simulink model "BatchEventsFor3StateMachines"  (R2021b)
settings: Solver=VariableStepAuto  StartTime=0.0  StopTime=10.0  RelTol=1e-3
model workspace (MATLAB code in the model file):
  | % Add the class folders into the path.
  | addpath model
  | addpath utils
  | 
  | %% Loading data from files.
  | % Data for supervisor 1.
  | utils1 = StateMachineUtils;
  | 
  | % From TCT: Load all events' number.
  | utils1 = utils1.loadEventsInAds('resources/tct/ALLEVENT.ADS');
  | 
  | % From TCT: Disabled events in each state.
  | utils1 = utils1.loadDisabledEventsInPdt('resources/tct/supervisor1/DATA_SIMSUP1_MG1.PDT');
  | 
  | % From TCT: Transition matrix.
  | utils1 = utils1.loadTransitionsInAds('resources/tct/supervisor1/SIMSUP1_MG1.ADS');
  | 
  | % Parameters for the block.
  | encodedStates1 = StateEncoder.encode(utils1.statesArray);
  | 
  | transitions1 = utils1.transitions;
  | 
  | allEvents1 = utils1.eventsArray;
  | 
  | % Data for supervisor 2.
  | utils2 = StateMachineUtils;
  | 
  | % From TCT: Load all events' number.
  | utils2 = utils2.loadEventsInAds('resources/tct/ALLEVENT.ADS');
  | 
  | % From TCT: Disabled events in each state.
  | utils2 = utils2.loadDisabledEventsInPdt('resources/tct/supervisor2/DATA_SIMSUP2_MG1.PDT');
  | 
  | % From TCT: Transition matrix.
  | utils2 = utils2.loadTransitionsInAds('resources/tct/supervisor2/SIMSUP2_MG1.ADS');
  | 
  | % Parameters for the block.
  | encodedStates2 = StateEncoder.encode(utils2.statesArray);
  | 
  | transitions2 = utils2.transitions;
  | 
  | allEvents2 = utils2.eventsArray;
  | 
  | % Data for supervisor 3.
  | utils3 = StateMachineUtils;
  | 
  | % From TCT: Load all events' number.
  | utils3 = utils3.loadEventsInAds('resources/tct/ALLEVENT.ADS');
  | 
  | % From TCT: Disabled events in each state.
  | utils3 = utils3.loadDisabledEventsInPdt('resources/tct/supervisor3/DATA_SIMSUP3_MG1.PDT');
  | 
  | % From TCT: Transition matrix.
  | utils3 = utils3.loadTransitionsInAds('resources/tct/supervisor3/SIMSUP3_MG1.ADS');
  | 
  | % Parameters for the block.
  | encodedStates3 = StateEncoder.encode(utils3.statesArray);
  | 
  | transitions3 = utils3.transitions;
  | 
  | allEvents3 = utils3.eventsArray;
settings Model: Creator=andrerangel  LastModifiedBy=andrerangel

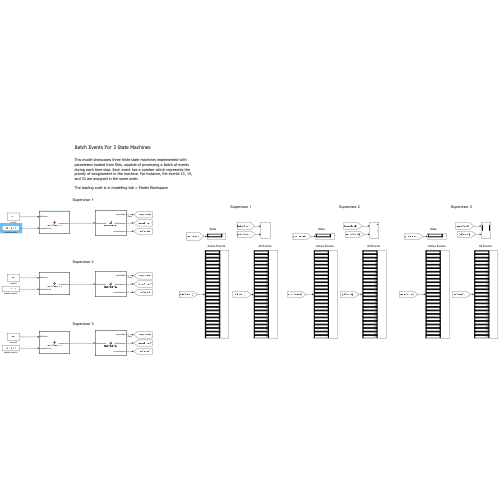
[thumbnail: Simulink's stored preview of the top-level diagram]
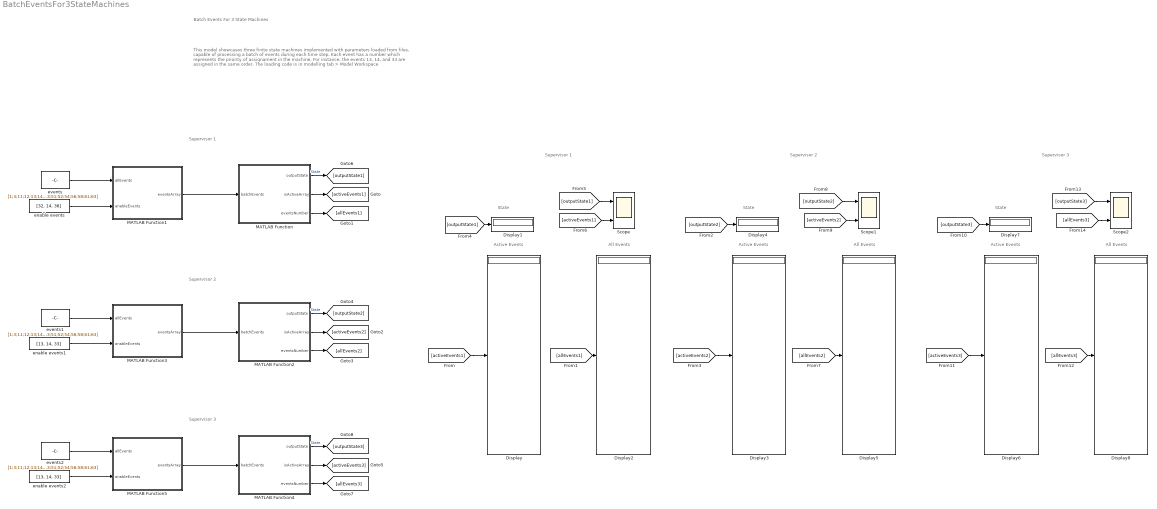
== system BatchEventsFor3StateMachines ==
  note: Active Events
  note: State
  note: This model showcases three finite state machines implemented with parameters loaded from files, capable of processing a batch of events during each time step. Each event has a number which represents the priority of assignament in the machine. For instance, the events 13, 14, and 33 are assigned in the same order.
      |
      | The loading code is in modelling tab > Model Workspace
  note: Supervisor 1
  note: All Events
  note: Batch Events For 3 State Machines
  note: All Events
  note: Supervisor 2
  note: Active Events
  note: State
  note: Supervisor 1
  note: All Events
  note: Supervisor 3
  note: Active Events
  note: State
  note: Supervisor 2
  note: Supervisor 3
  Display{,1..8} (9 alike) : Display
  MATLAB Function : MATLAB Function  TreatAsAtomicUnit=on
  MATLAB Function1 : MATLAB Function  TreatAsAtomicUnit=on
  MATLAB Function2 : MATLAB Function  TreatAsAtomicUnit=on
  MATLAB Function3 : MATLAB Function  TreatAsAtomicUnit=on
  MATLAB Function4 : MATLAB Function  TreatAsAtomicUnit=on
  MATLAB Function5 : MATLAB Function  TreatAsAtomicUnit=on
  Scope : Scope  NumInputPorts=2
  Scope1 : Scope  NumInputPorts=2
  Scope2 : Scope  NumInputPorts=2
  enable events : Constant  Value=[32, 14, 36]
  enable events1 : Constant  Value=[13, 14, 33]
  enable events2 : Constant  Value=[13, 14, 33]
  events : Constant  Value=[1;3;11;12;13;14;16;21;23;25;27;31;32;33;34;36;41;43;51;52;54;56;58;61;63]
  events1 : Constant  Value=[1;3;11;12;13;14;16;21;23;25;27;31;32;33;34;36;41;43;51;52;54;56;58;61;63]
  events2 : Constant  Value=[1;3;11;12;13;14;16;21;23;25;27;31;32;33;34;36;41;43;51;52;54;56;58;61;63]
  wires:
  MATLAB Function1/1(eventsArray) -> MATLAB Function/1(batchEvents)
  [allEvents1] -> Display2/1
  [outputState2] -> Scope1/1
  [allEvents2] -> Display5/1
  [activeEvents2] -> Scope1/2
  [activeEvents2] -> Display3/1
  MATLAB Function/1(outputState) -> [outputState1]  "State"
  enable events/1 -> MATLAB Function1/2(anableEvents)
  [outputState1] -> Display1/1
  events/1 -> MATLAB Function1/1(allEvents)
  [activeEvents1] -> Scope/2
  [outputState1] -> Scope/1
  [outputState2] -> Display4/1
  MATLAB Function/2(isActiveArray) -> [activeEvents1]
  [activeEvents1] -> Display/1
  MATLAB Function/3(eventsNumber) -> [allEvents1]
  MATLAB Function2/3(eventsNumber) -> [allEvents2]
  MATLAB Function2/2(isActiveArray) -> [activeEvents2]
  events1/1 -> MATLAB Function3/1(allEvents)
  enable events1/1 -> MATLAB Function3/2(anableEvents)
  MATLAB Function2/1(outputState) -> [outputState2]  "State"
  MATLAB Function3/1(eventsArray) -> MATLAB Function2/1(batchEvents)
  MATLAB Function5/1(eventsArray) -> MATLAB Function4/1(batchEvents)
  MATLAB Function4/1(outputState) -> [outputState3]  "State"
  enable events2/1 -> MATLAB Function5/2(anableEvents)
  events2/1 -> MATLAB Function5/1(allEvents)
  MATLAB Function4/2(isActiveArray) -> [activeEvents3]
  MATLAB Function4/3(eventsNumber) -> [allEvents3]
  [outputState3] -> Display7/1
  [activeEvents3] -> Display6/1
  [allEvents3] -> Scope2/2
  [allEvents3] -> Display8/1
  [outputState3] -> Scope2/1

== matlab function BatchEventsFor3StateMachines/MATLAB Function1 ==
  data: allEvents input; anableEvents input; eventsArray output
function eventsArray = eventsGenerator(allEvents, anableEvents)

[~, indexes] = ismember(anableEvents, allEvents);

eventsArray = zeros(length(allEvents), 1);

eventsArray(indexes) = 1;

== matlab function BatchEventsFor3StateMachines/MATLAB Function ==
  data: batchEvents input; outputState output size=[1 1]; isActiveArray output; eventsNumber output; allEvents1 parameter; transitions1 parameter; encodedStates1 parameter
function [outputState, isActiveArray, eventsNumber] = stateMachine1( ...
    batchEvents, ...
    allEvents1, ...
    transitions1, ...
    encodedStates1)
% State Machine with parameters from files.
% Receives a batch of events and process one event at time, starting with
% the event of index 1.
% batchEvents: array with 0s and 1s where 1 is the enabled event while 0,
% is disabled event;
% allEvents: numbers of the events;
% transitions: matrix of transitions;
% encodedStates: Encoded states array to be decoded before the pass it to
% StateMachines as an argument.

% Initialize a persistent object. Its value will not be erased as this
% block finishes.
persistent stateMachine

% Assign the persistent object to the StateMachine class with data passed
% as parameters.
if (isempty(stateMachine))
    statesArray = StateEncoder.decode(encodedStates1);                        
    stateMachine = StateMachine(statesArray, transitions1, allEvents1);
end

anabledEvents = allEvents1(logical(batchEvents));

% loop through an array of events:
for i=1:length(anabledEvents)
    stateMachine.inputEvent = anabledEvents(i);
end
outputState = stateMachine.currentState.number;
isActiveArray = stateMachine.currentState.activeEvents;
eventsNumber = stateMachine.eventsArray;

== matlab function BatchEventsFor3StateMachines/MATLAB Function2 ==
  data: batchEvents input; outputState output size=[1 1]; isActiveArray output; eventsNumber output; allEvents2 parameter; transitions2 parameter; encodedStates2 parameter
function [outputState, isActiveArray, eventsNumber] = stateMachine2( ...
    batchEvents, ...
    allEvents2, ...
    transitions2, ...
    encodedStates2)
% State Machine with parameters from files.
% Receives a batch of events and process one event at time, starting with
% the event of index 1.
% batchEvents: array with 0s and 1s where 1 is the enabled event while 0,
% is disabled event;
% allEvents: numbers of the events;
% transitions: matrix of transitions;
% encodedStates: Encoded states array to be decoded before the pass it to
% StateMachines as an argument.

% Initialize a persistent object. Its value will not be erased as this
% block finishes.
persistent stateMachine

% Assign the persistent object to the StateMachine class with data passed
% as parameters.
if (isempty(stateMachine))
    statesArray = StateEncoder.decode(encodedStates2);                        
    stateMachine = StateMachine(statesArray, transitions2, allEvents2);
end

anabledEvents = allEvents2(logical(batchEvents));

% loop through an array of events:
for i=1:length(anabledEvents)
    stateMachine.inputEvent = anabledEvents(i);
end
outputState = stateMachine.currentState.number;
isActiveArray = stateMachine.currentState.activeEvents;
eventsNumber = stateMachine.eventsArray;

== matlab function BatchEventsFor3StateMachines/MATLAB Function3 ==
  data: allEvents input; anableEvents input; eventsArray output
function eventsArray = eventsGenerator(allEvents, anableEvents)

[~, indexes] = ismember(anableEvents, allEvents);

eventsArray = zeros(length(allEvents), 1);

eventsArray(indexes) = 1;

== matlab function BatchEventsFor3StateMachines/MATLAB Function4 ==
  data: batchEvents input; outputState output size=[1 1]; isActiveArray output; eventsNumber output; allEvents3 parameter; transitions3 parameter; encodedStates3 parameter
function [outputState, isActiveArray, eventsNumber] = stateMachine3( ...
    batchEvents, ...
    allEvents3, ...
    transitions3, ...
    encodedStates3)
% State Machine with parameters from files.
% Receives a batch of events and process one event at time, starting with
% the event of index 1.
% batchEvents: array with 0s and 1s where 1 is the enabled event while 0,
% is disabled event;
% allEvents: numbers of the events;
% transitions: matrix of transitions;
% encodedStates: Encoded states array to be decoded before the pass it to
% StateMachines as an argument.

% Initialize a persistent object. Its value will not be erased as this
% block finishes.
persistent stateMachine

% Assign the persistent object to the StateMachine class with data passed
% as parameters.
if (isempty(stateMachine))
    statesArray = StateEncoder.decode(encodedStates3);                        
    stateMachine = StateMachine(statesArray, transitions3, allEvents3);
end

anabledEvents = allEvents3(logical(batchEvents));

% loop through an array of events:
for i=1:length(anabledEvents)
    stateMachine.inputEvent = anabledEvents(i);
end
outputState = stateMachine.currentState.number;
isActiveArray = stateMachine.currentState.activeEvents;
eventsNumber = stateMachine.eventsArray;

== matlab function BatchEventsFor3StateMachines/MATLAB Function5 ==
  data: allEvents input; anableEvents input; eventsArray output
function eventsArray = eventsGenerator(allEvents, anableEvents)

[~, indexes] = ismember(anableEvents, allEvents);

eventsArray = zeros(length(allEvents), 1);

eventsArray(indexes) = 1;
